simulink model "system_model"  (R2024a)
settings: Solver=VariableStepAuto  StartTime=0.0  StopTime=100000.0  MaxStep=1  RelTol=1e-9
values from neighbouring files (symbols this model uses):
  a_leader = 500*10^3 + earth_radi    (= 6871000)    [main.m]    (also in main_2.m)
  B_f_max = (C_d*A_f_max)/m_f    (= 0.78)    [main_2.m]
  B_f_min = (C_d*A_f_min)/m_f    (= 0.13)    [main_2.m]
  B_l_max = (C_d*A_l_max)/m_l    (= 0.78)    [main_2.m]
  B_l_min = (C_d*A_l_min)/m_l    (= 0.13)    [main_2.m]
  earth_radi = 6371*10^3    (= 6371000)    [main.m]    (also in main_2.m)
  J = eye(3)    [attitude.m]    (also in state_func.m = 43943563035.8; state_func_test.m = J_2 * R_E^2)
  J_2 = 1.08263 * 10^(-3)    (= 0.00108263)    [main.m]    (also in main_2.m; state_func.m)
  Kd = 5    [attitude.m]
  Kp = 5    [attitude.m]
  m_f = 1    [main.m]    (also in main_2.m = 2)
  m_l = 1    [main.m]    (also in main_2.m = 2)
  mu = 13/ 26.98    (= 0.481838398814)    [drag_coefficent_ruff_estimation.m]    (also in main.m = 6.67e-11; main_2.m = 398589196000000; state_func.m = 398589196000000; untitled5.m)
  q_0 = q_0 /norm(q_0)    [attitude.m]
  rho_leader = mean_rho_500km    (= 7.3e-13)    [main_2.m]
  w_0 = [1; 2; 1]    [attitude.m]
  x = theta_vec    [drag_coefficent_ruff_estimation.m]    (also in main.m = [d_a; d_lambda; d_e_x; d_e_y; d_i_x; d_i_y; d_Ballistic]; main_2.m = [d_a; d_lambda; d_e_x; d_e_y; d_i_x; d_i_y])
  x_f_prop = [a_follower; m_follower; e_follower; omega_follower; Omega_follower; i_follower]    [main_2.m]
  x_l_prop = [a_leader; m_leader; e_leader; omega_leader; Omega_leader; i_leader]    [main_2.m]
libraries: mpclib x1, slpidlib x1
(part 2 of 2)

== matlab function system_model/orbit_Propegation/MATLAB Function5 ==
  data: oeosc input; oemean output; j2 input; req input
function oemean = osc2mean (oeosc, j2, req)

% convert osculating classical orbital elements
% to mean classical orbital elements

% input

%  oeosc(1) = osculating semimajor axis (kilometers)
%  oeosc(2) = osculating orbital eccentricity (non-dimensional)
%             (0 <= eccentricity < 1)
%  oeosc(3) = osculating orbital inclination (radians)
%             (0 <= inclination <= pi)
%  oeosc(4) = osculating argument of perigee (radians)
%             (0 <= argument of perigee <= 2 pi)
%  oeosc(5) = osculating right ascension of ascending node (radians)
%             (0 <= raan <= 2 pi)
%  oeosc(6) = osculating true anomaly (radians)
%             (0 <= true anomaly <= 2 pi)

% output

%  oemean(1) = mean semimajor axis (kilometers)
%  oemean(2) = mean orbital eccentricity (non-dimensional)
%              (0 <= eccentricity < 1)
%  oemean(3) = mean orbital inclination (radians)
%              (0 <= inclination <= pi)
%  oemean(4) = mean argument of perigee (radians)
%              (0 <= argument of perigee <= 2 pi)
%  oemean(5) = mean right ascension of ascending node (radians)
%              (0 <= raan <= 2 pi)
%  oemean(6) = mean true anomaly (radians)
%              (0 <= true anomaly <= 2 pi)

% Orbital Mechanics with MATLAB

%%%%%%%%%%%%%%%%%%%%%%%%%%%%%%%

%global req j2

pi2 = 2.0 * pi;

oetmp = zeros(6, 1);

for i = 1:1:6
    
    oetmp(i) = oeosc(i);
    
end

a = sin(oetmp(6)) * sqrt(1.0 - oetmp(2) * oetmp(2));

b = oetmp(2) + cos(oetmp(6));

% eccentric anomaly

eanom = atan3(a, b);

% mean anomaly

oetmp(6) = mod(eanom - oetmp(2) * sin(eanom), pi2);

aos = oetmp(1);
eos = oetmp(2);
ios = oetmp(3);
apos = oetmp(4);
ranos = oetmp(5);
maos = oetmp(6);

aa = 1.0 / 3.0 - 0.5 * sin(ios)^2;

bb = 0.5 * sin(ios)^2;

if (eos < 0.01)
    
    lamos = mod(maos + apos, pi2);
    
    zos = eos * cos(apos);
    
    etaos = eos * sin(apos);
    
    sl = sin(lamos);
    cl = cos(lamos);
    
    s2l = sin(2 * lamos);
    c2l = cos(2 * lamos);
    
    s3l = sin(3 * lamos);
    c3l = cos(3 * lamos);
    
    s4l = sin(4 * lamos);
    c4l = cos(4 * lamos);
    
    s2i = sin(2 * ios);
    
    ci = cos(ios);
    
    am = aos;
    im = ios;
    ranm = ranos;
    mam = maos;
    lamm = lamos;
    zm = zos;
    etam = etaos;
    
    for n = 1:1:5
        
        asp = 3 * j2 * req * req / am * (bb * c2l + (1 - 3.5 * bb) ...
            * zm * cl + (1 - 2.5 * bb) * etam * sl + 3.5 * bb ...
            * (zm * c3l + etam * s3l));
        
        am = aos-asp;
        
        isp = 3 * j2 / 8 * req * req / am^2 * s2i * (c2l - zm * cl ...
            + etam * sl + 7/3 * (zm * c3l + etam * s3l));
        
        im = ios - isp;
        
        ci = cos(im);
        
        s2i = sin(2 * im);
        
        bb = 0.5 * sin(im)^2;
        
        ransp = 1.5 * j2 * req * req / am^2 * ci ...
            * (0.5 * s2l - 3.5 * zm * sl + 2.5 * etam * cl ...
            + 7/6 * (zm * s3l - etam * c3l));
        
        ranm = ranos - ransp;
        
        lamsp = 1.5 * j2 * req * req / (am * am) ...
            * (-0.5 * (1 - 5 * bb) * s2l + (7 - 77/4 * bb) ...
            * zm * sl - (6 - 55/4 * bb) * etam * cl - (7/6 - 77/12 * bb) ...
            * (zm * s3l - etam * c3l));
        
        lamm = lamos - lamsp;
        
        sl = sin(lamm);
        cl = cos(lamm);
        s2l = sin(2*lamm);
        c2l = cos(2*lamm);
        s3l = sin(3*lamm);
        c3l = cos(3*lamm);
        s4l = sin(4*lamm);
        c4l = cos(4*lamm);
        
        zsp = 1.5 * j2 * req * req / am^2 * ((1 - 2.5 * bb) * cl ...
            + 7/6 * bb * c3l + (1.5 - 5 * bb) * zm * c2l + (2 - 3 * bb) ...
            * etam * s2l + 17/4 * bb * (zm * c4l + etam * s4l));
        
        zm = zos - zsp;
        
        etasp = 1.5 * j2 * req * req / am^2 * ((1 - 3.5 * bb) * sl ...
            + 7/6 * bb * s3l + (1 - 6 * bb) * zm * s2l - (1.5 - 4 * bb) ...
            * etam * c2l + 17/4 * bb * (zm * s4l - etam * c4l));
        
        etam = etaos - etasp;
    end
    
    em = sqrt(etam^2 + zm^2);
    
    apm = 0;
    
    if (em > 1.0e-8)
        
        apm = atan2(etam, zm);
        
    end
    
    % "mean" mean anomaly
    
    mam = mod(lamm - apm, pi2);
    
else
    
    pm = aos*(1-eos^2);
    am = aos;
    em = eos;
    im = ios;
    apm = apos;
    ranm = ranos;
    mam = maos;
    
    [~, tam] = kepler1(mam, em);
    
    um = mod(apm+tam, pi2);
    
    hm = pm/(1+em*cos(tam));
    
    for n = 1:1:5
        
        asp = 3*j2*req*req/am*((am/hm)^3*(aa+bb*cos(2*um)) ...
            -aa*(1-em^2)^(-1.5));
        
        am = aos-asp;
        
        isp = 3/8*j2*req^2/pm^2*sin(2*im)*(cos(2*um) ...
            +em*cos(tam+2*apm)+1/3*em*cos(3*tam+2*apm));
        
        im = ios-isp;
        
        aa = 1/3-0.5*sin(im)^2;
        
        bb = 0.5*sin(im)^2;
        
        esp = 1.5*j2*req*req/am^2*((1-em^2)/em*((am/hm)^3 ...
            *(aa+bb*cos(2*um))-aa*(1-em^2)^(-1.5))-bb/(em*(1-em^2)) ...
            *(cos(2*um)+em*cos(tam+2*apm)+em*cos(3*tam+2.*apm)/3));
        
        em = eos-esp;
        
        pm = am * (1.0 - em^2);
        
        hm = pm / (1.0 + em * cos(tam));
        
        tam = mod(tam, 2.0 * pi);
        
        mam = mod(mam, 2.0 * pi);
        
        if ((abs(tam-pi) <= 1.0e-06) || (abs(mam-pi) <= 1.0e-06) || ...
                (abs(tam) <= 1.0e-06) || (abs(mam) <= 1.0e-06))
            
            eqoc = 0;
            
        else
            
            eqoc = tam-mam;
            
        end
        
        ransp = -1.5*j2*(req/pm)^2*cos(im)*(eqoc+em*sin(tam) ...
            -0.5*sin(2*um)-0.5*em*sin(tam+2*apm)-1/6*em*sin(3*tam+2*apm));
        
        ranm = ranos-ransp;
        
        apsp = 1.5*j2*(req/pm)^2*((2-5*bb)*(eqoc+em*sin(tam)) ...
            +(1-3*bb)*((1-0.25*em*em)*sin(tam)/em+0.5*sin(2*tam) ...
            +em*sin(3*tam)/12)-(0.5*bb+(0.5-15/8*bb)*em^2)/em*sin(tam+2*apm) ...
            +em/8*bb*sin(tam-2*apm)-0.5*(1-5*bb)*sin(2*um)+(7/6*bb ...
            -1/6*em^2*(1-19/4*bb))/em*sin(3*tam+2*apm) ...
            +0.75*bb*sin(4*tam+2*apm)+em/8*bb*sin(5*tam+2*apm));
        
        apm = apos-apsp;
        
        masp = 1.5*j2*(req/pm)^2*sqrt(1-em^2)/em*(-(1-3*bb)*((1-em^2/4) ...
            *sin(tam)+em/2*sin(2*tam)+em^2/12*sin(3*tam)) ...
            +bb*(0.5*(1+1.25*em^2)*sin(tam+2*apm)-em^2/8*sin(tam-2*apm) ...
            -7/6*(1-em^2/28)*sin(3*tam+2*apm)-0.75*em*sin(4*tam+2*apm) ...
            -em^2/8*sin(5*tam+2*apm)));
        
        mam = maos-masp;
        
        [~, tam] = kepler1(mam, em);
        
        um = mod(apm + tam, pi2);
    end
end
oemean = zeros(7,1);
oemean(1) = am;
oemean(2) = em;
oemean(3) = im;
oemean(4) = mod(apm, pi2);
oemean(5) = mod(ranm, pi2);
oemean(6) = mod(mam, pi2);

[~, ta] = kepler1(oemean(6), em);

oemean(7) = ta;


end

function y = atan3 (a, b)

% four quadrant inverse tangent

% input

%  a = sine of angle
%  b = cosine of angle

% output

%  y = angle (radians; 0 =< c <= 2 * pi)

% Orbital Mechanics with MATLAB

%%%%%%%%%%%%%%%%%%%%%%%%%%%%%%%

epsilon = 0.0000000001;

pidiv2 = 0.5 * pi;

if (abs(a) < epsilon)
    y = (1 - sign(b)) * pidiv2;
    return;
else
    c = (2 - sign(a)) * pidiv2;
end

if (abs(b) < epsilon)
    y = c;
    return;
else
    y = c + sign(a) * sign(b) * (abs(atan(a / b)) - pidiv2);
end

end

function [eanom, tanom] = kepler1 (manom, ecc)

% solve Kepler's equation for circular,
% elliptic and hyperbolic orbits

% Danby's method

% input

%  manom = mean anomaly (radians)
%  ecc   = orbital eccentricity (non-dimensional)

% output

%  eanom = eccentric anomaly (radians)
%  tanom = true anomaly (radians)

% Orbital Mechanics with MATLAB

%%%%%%%%%%%%%%%%%%%%%%%%%%%%%%%

%global  niter

% define convergence criterion

ktol = 1.0e-10;

pi2 = 2.0 * pi;

xma = manom - pi2 * fix(manom/pi2);

% initial guess

if (ecc == 0.0)
    
    % circular orbit

    tanom = xma;
    eanom = xma;
    return;
    
elseif (ecc < 1.0)
    % elliptic orbit

    eanom = xma + 0.85 * sign(sin(xma)) * ecc;

else
    % hyperbolic orbit

    eanom = log(2.0 * xma / ecc + 1.8);
end

% perform iterations

niter = 0;

while(1)
    
    if (ecc < 1)

        % elliptic orbit

        s = ecc * sin(eanom);
        c = ecc * cos(eanom);

        f = eanom - s - xma;
        fp = 1 - c;
        fpp = s;
        fppp = c;
        
    else

        % hyperbolic orbit

        s = ecc * sinh(eanom);
        c = ecc * cosh(eanom);

        f = s - eanom - xma;
        fp = c - 1;
        fpp = s;
        fppp = c;
        
    end

    niter = niter + 1;

    % check for convergence

    if (abs(f) <= ktol || niter > 20)
        
        break;
        
    end

    % update eccentric anomaly

    delta = -f / fp;

    deltastar = -f / (fp + 0.5 * delta * fpp);

    deltak = -f / (fp + 0.5 * deltastar * fpp ...
        + deltastar * deltastar * fppp / 6);

    eanom = eanom + deltak;
end

if (niter > 20)
    
    %clc; home;
    
    fprintf('\n\n   more than 20 iterations in kepler1 \n\n');
    
    %pause;
    
    %return;
end

% compute true anomaly

if (ecc < 1)
    % elliptic orbit

    sta = sqrt(1 - ecc * ecc) * sin(eanom);
    cta = cos(eanom) - ecc;
else
    % hyperbolic orbit

    sta = sqrt(ecc * ecc - 1) * sinh(eanom);
    cta = ecc - cosh(eanom);
end

tanom = atan3(sta, cta);


end

== matlab function system_model/g(x) ==
  data: u input; x input; g_x output; x_f input; rho input
function g_x = g(u, x, x_f, rho)
%Note that these equations have elliminated the need for leader spacecraft
%orbit properties

B   = u(1);
B_f = u(2);

rho_c = rho;


a_c = x_f(1);
%u_c = x_f(2);
e_c = x_f(2);
% e_c = x_f(3); - not corrrect here
%i_c = x_f(4);  - not correct here
i_c = x_f(3);
omega_c = x_f(4);
Omega_c = x_f(5);
Nu_c    = x_f(6);
%  oemean(1) = mean semimajor axis (kilometers)
%  oemean(2) = mean orbital eccentricity (non-dimensional)
%              (0 <= eccentricity < 1)
%  oemean(3) = mean orbital inclination (radians)
%              (0 <= inclination <= pi)
%  oemean(4) = mean argument of perigee (radians)
%              (0 <= argument of perigee <= 2 pi)
%  oemean(5) = mean right ascension of ascending node (radians)
%              (0 <= raan <= 2 pi)
%  oemean(6) = mean true anomaly (radians)
%              (0 <= true anomaly <= 2 pi)
%x_f = [a_dot; M_dot; e_dot; omega_dot; Omega_dot; i_dot];

betta   = B*f(e_c)*rho;
betta_c = B_f *f(e_c) * rho_c;
E       = sqrt(e_c^2 + x(3)^2 + x(4)^2 - 2*e_c*(x(3)*cos(omega_c) + x(4)*sin(omega_c)));



g_x = zeros(6,1);

g_x(1) = (1 + x(1))*(betta_c/(1-e_c) + betta/(E-1) );
g_x(2) = 0;
g_x(3) = betta_c * cos(omega_c) + E^-1 * betta*( x(3) - e_c*cos(omega_c));
g_x(4) = betta_c * sin(omega_c) + E^-1 * betta*( x(4) - e_c*sin(omega_c));
g_x(5) = 0;
g_x(6) = 0;

end
     
function f = f(e)
    f = 1.61*10^4*e^0.02701 -1.61*10^4;
end

== matlab function system_model/orbit_Propegation/MATLAB Function6 ==
  data: xn output; x input
function xn = kozsak(x)

iflag = 2;

% convert between osculating and mean classical orbital elements

% method due to Chauncey Uphoff (JPL IOM 312/85.2-927)

% input

%  iflag = 1 => mean to osculating
%          2 => osculating to mean

%  x = osculating or mean orbital elements

% output

%  xn = osculating or mean orbital elements

% Orbital Mechanics with MATLAB

%%%%%%%%%%%%%%%%%%%%%%%%%%%%%%%

pi2 = 2.0 * pi;

xi = zeros(6, 1);

xn = zeros(6, 1);

% set max iterations based on input orbital eccentricity x(2)

if (x(2) < 0.1)
    
    imax = 10;
    
elseif (x(2) < 0.01)
    
    imax = 20;
    
elseif (x(2) < 0.001)
    
    imax = 30;
    
else
    
    imax = 5;
    
end

for i = 1:1:6
    
    xi(i) = x(i);
    
end

icount = 0;

while (1)
    
    % compute periodics
    
    dx = delm(x);
    
    if (iflag == 2)
        
        % osculating to mean
        
        icount = icount + 1;
        
        for i = 1:1:6
            
            xn(i) = xi(i) - dx(i);
            
        end
        
        % check for negative eccentricity
        
        if (xn(2) < 0.0)
            
            xn(2) = 0.0;
            
        end
        
        for i = 3:1:6
            
            xn(i) = mod(xn(i) + pi2, pi2);
            
        end
        
        % check for maximum iterations
        
        if (icount == imax)
            
            break;
            
        end
        
        % load mean orbital elements
        
        for i = 1:1:6
            
            x(i) = xn(i);
            
        end
        
    else
        
        % mean to osculating
        
        for i = 1:1:6
            
            xn(i) = xi(i) + dx(i);
            
        end
        
        for i = 3:1:6
            
            xn(i) = mod(xn(i) + pi2, pi2);
            
        end
        
        break;
        
    end
    
end

end

function dx = delm (x)

% compute [osculating - mean] classical orbital elements

% input

%  x = mean classical orbital elements

% output

%  dx = [osculating - mean] classical orbital elements

% Orbital Mechanics with MATLAB

%%%%%%%%%%%%%%%%%%%%%%%%%%%%%%%

mu  = 98600.4415;
req = 6378.14;
xj2 = 0.001082634;

pi2 = 2.0 * pi;

dx = zeros(6, 1);

% semimajor axis (kilometers)

a = x(1);

% orbital eccentricity (non-dimensional)

e = x(2);

% orbital inclination (radians)

ai = x(3);

% right ascension of the ascending node (radians)

an = x(4);

% argument of perigee (radians)

w = x(5);

% mean anomaly (radians)

am = x(6);

% compute true anomaly from mean anomaly

f = anomly(2, am, e);

f = mod(f + pi2, pi2);

am = mod(am + pi2, pi2);

si = sin(ai);
ci = cos(ai);
ti = si / ci;

si2 = si * si;
ci2 = ci * ci;

sf = sin(f);
cf = cos(f);
s2f = sin(2.0 * f);

u = f + w;
e2 = e * e;
esf = e * sf;

d1 = 1.0 - e2;
d2 = sqrt(d1);
d3 = e * cf;
d4 = 1.0 + d3;
d42 = d4 * d4;
d5 = 1.0 + d2;
d6 = (3.0 * ci2 - 1.0) / d5;

p = a * d1;

d7 = sqrt(mu / p);

r = p / d4;

rdot = d7 * esf;

twou = 2.0 * u;

twow = 2.0 * w;

s2u = sin(twou);
c2u = cos(twou);

sf2w = sin(f + twow);

d8 = 3.0 * f + twow;

s3f2w = sin(d8);
cf2w = cos(f + twow);
c3f2w = cos(d8);

q1 = xj2 * (req / p) ^ 2;

di = 0.75 * q1 * si * ci * (c2u + e * cf2w + e / 3.0 * c3f2w);

dp = 2.0 * p * ti * di;

dummy1 = f - am + esf - 0.5 * s2u - 0.5 * e * sf2w - e * s3f2w / 6.0;

dn = -1.5 * q1 * ci * dummy1;

dr = -0.25 * p * q1 * ((3.0 * ci2 - 1.0) * (2.0 * d2 / d4 + d3 / d5 + 1.0) - si2 * c2u);

drdot = 0.25 * d7 * q1 * (d6 * esf * (d2 * d5 + d42) - 2.0 * si2 * d42 * s2u);

du = -0.125 * q1 * (6.0 * (1.0 - 5.0 * ci2) * (f - am) + 4.0 * esf * ((1.0 - 6.0 * ci2) ...
    - d6) - d6 * e2 * s2f + 2.0 * (5.0 * ci2 - 2.0) * e * sf2w + (7.0 * ci2 - 1.0) ...
    * s2u + 2.0 * ci2 * e * s3f2w);

pnw = p + dp;

ainw = ai + di;

annw = an + dn;

rnw = r + dr;

rdotnw = rdot + drdot;

unw = u + du;

aa = pnw / rnw - 1.0;

bb = sqrt(pnw / mu) * rdotnw;

enw2 = aa * aa + bb * bb;

enw = sqrt(enw2);

fnw = atan2(bb, aa);

anw = pnw / (1.0 - enw2);

wnw = unw - fnw;

amnw = anomly(5, fnw, enw);

%  compute [osculating - mean] classical orbital elements

dx(1) = anw - a;

dx(2) = enw - e;

dx(3) = ainw - ai;

dx(4) = annw - an;

dx(5) = wnw - w;

dx(6) = amnw - am;

end

function aout = anomly(nflag, ain, ecc)

% orbital anomaly function

% input

%  nflag = 1 => mean to eccentric
%          2 => mean to true
%          3 => eccentric to mean
%          4 => eccentric to true
%          5 => true to mean
%          6 => true to eccentric

%  ain = input anomaly (radians)
%  ecc = orbital eccentricity

% output

%  aout = output anomaly (radians)

% Orbital Mechanics with MATLAB

%%%%%%%%%%%%%%%%%%%%%%%%%%%%%%%

switch nflag
    
    case {1, 2}
        
        % mean anomaly
        
        am = ain;
        
    case {3, 4}
        
        % eccentric anomaly
        
        ea = ain;
        
    case {5, 6}
        
        % true anomaly
        
        f = ain;
        
end

if (nflag == 1 || nflag == 2)
    
    % eccentric anomaly (radians)
    
    ea = kepler(am, ecc);
    
end

if (nflag == 2 || nflag == 4)
    
    % true anomaly (radians)
    
    f = 2.0 * atan(sqrt((1.0 + ecc) / (1.0 - ecc)) * tan(ea / 2.0));
    
end

if (nflag == 5 || nflag == 6)
    
    % eccentric anomaly (radians)
    
    ea = 2.0 * atan(sqrt((1.0 - ecc) / (1.0 + ecc)) * tan(f / 2.0));
    
end

if (nflag == 5 || nflag == 3)
    
    % mean anomaly (radians)
    
    am = ea - ecc * sin(ea);
    
end

switch nflag
    
    case {1, 6}
        
        % eccentric anomaly
        
        aout = ea;
        
    case {2, 4}
        
        % true anomaly
        
        aout = f;
        
    case {3, 5}
        
        % mean anomaly
        
        aout = am;
end
end


function eanom = kepler(manom, ecc)

% solve Kepler's equation for circular,
% elliptic and hyperbolic orbits

% Danby's method

% input

%  manom = mean anomaly (radians)
%  ecc   = orbital eccentricity (non-dimensional)

% output

%  eanom = eccentric anomaly (radians)

% Orbital Mechanics with MATLAB

%%%%%%%%%%%%%%%%%%%%%%%%%%%%%%%

% define convergence criterion

ktol = 1.0e-10;

pi2 = 2.0 * pi;

xma = manom - pi2 * fix(manom/pi2);

% initial guess

if (ecc == 0.0)
    
    % circular orbit
    
    eanom = xma;
    
    return;
    
elseif (ecc < 1.0)
    
    % elliptic orbit

    eanom = xma + 0.85 * sign(sin(xma)) * ecc;

else
    
    % hyperbolic orbit

    eanom = log(2.0 * xma / ecc + 1.8);
    
end

% perform iterations

niter = 0;

while(1)
    
    if (ecc < 1.0)

        % elliptic orbit

        s = ecc * sin(eanom);
        c = ecc * cos(eanom);

        f = eanom - s - xma;
        fp = 1.0 - c;
        fpp = s;
        fppp = c;
        
    else

        % hyperbolic orbit

        s = ecc * sinh(eanom);
        c = ecc * cosh(eanom);

        f = s - eanom - xma;
        fp = c - 1.0;
        fpp = s;
        fppp = c;
        
    end

    niter = niter + 1;

    % check for convergence

    if (abs(f) <= ktol || niter > 20)
        
        break;
        
    end

    % update eccentric anomaly

    delta = -f / fp;

    deltastar = -f / (fp + 0.5 * delta * fpp);

    deltak = -f / (fp + 0.5 * deltastar * fpp ...
        + deltastar * deltastar * fppp / 6.0);

    eanom = eanom + deltak;
    
end

if (niter > 20)
    
    fprintf('\n\n   more than 20 iterations in kepler \n\n');

end






end

== matlab function system_model/orbit_Propegation/MATLAB Function7 ==
  data: x_f input; x_l input; d_a output; d_lambda output; d_e_x output; d_e_y output; d_i_x output; d_i_y output
function [d_a, d_lambda, d_e_x, d_e_y, d_i_x, d_i_y] = toRelOribtialElements(x_f, x_l)


a_f     = x_f(1);
e_f     = x_f(2);
i_f     = x_f(3);
omega_f = x_f(4);
Omega_f = x_f(5);
M_f     = x_f(6);

a_l     = x_l(1);
e_l     = x_l(2);
i_l     = x_l(3);
omega_l = x_l(4);
Omega_l = x_l(5);
M_l     = x_l(6);



u_l    = omega_l + M_l;
u_f    = omega_f + M_f;
u_diff =  ssa(M_f -M_l) + ssa(omega_f - omega_l); 

d_a          = (a_f - a_l) / a_l;
%d_lambda     = (u_f - u_l) + (Omega_f - Omega_l)*cos(i_l);
d_lambda     = u_diff + (Omega_f - Omega_l)*cos(i_l);
d_e_x        = e_f*cos(omega_f) - e_l*cos(omega_l);
d_e_y        = e_f*sin(omega_f) - e_l*sin(omega_l);
d_i_x        = i_f - i_l;
d_i_y        = (Omega_f -Omega_l)*sin(i_l);


end

function angle = ssa(angle)
    angle = mod( angle + pi, 2 * pi ) - pi; 
end

== matlab function system_model/orbit_Propegation/MATLAB Function8 ==
  data: oeosc input; oemean output; j2 input; req input
function oemean = osc2mean (oeosc, j2, req)

% convert osculating classical orbital elements
% to mean classical orbital elements

% input

%  oeosc(1) = osculating semimajor axis (kilometers)
%  oeosc(2) = osculating orbital eccentricity (non-dimensional)
%             (0 <= eccentricity < 1)
%  oeosc(3) = osculating orbital inclination (radians)
%             (0 <= inclination <= pi)
%  oeosc(4) = osculating argument of perigee (radians)
%             (0 <= argument of perigee <= 2 pi)
%  oeosc(5) = osculating right ascension of ascending node (radians)
%             (0 <= raan <= 2 pi)
%  oeosc(6) = osculating true anomaly (radians)
%             (0 <= true anomaly <= 2 pi)

% output

%  oemean(1) = mean semimajor axis (kilometers)
%  oemean(2) = mean orbital eccentricity (non-dimensional)
%              (0 <= eccentricity < 1)
%  oemean(3) = mean orbital inclination (radians)
%              (0 <= inclination <= pi)
%  oemean(4) = mean argument of perigee (radians)
%              (0 <= argument of perigee <= 2 pi)
%  oemean(5) = mean right ascension of ascending node (radians)
%              (0 <= raan <= 2 pi)
%  oemean(6) = mean true anomaly (radians)
%              (0 <= true anomaly <= 2 pi)

% Orbital Mechanics with MATLAB

%%%%%%%%%%%%%%%%%%%%%%%%%%%%%%%

%global req j2

pi2 = 2.0 * pi;

oetmp = zeros(6, 1);

for i = 1:1:6
    
    oetmp(i) = oeosc(i);
    
end

a = sin(oetmp(6)) * sqrt(1.0 - oetmp(2) * oetmp(2));

b = oetmp(2) + cos(oetmp(6));

% eccentric anomaly

eanom = atan3(a, b);

% mean anomaly

oetmp(6) = mod(eanom - oetmp(2) * sin(eanom), pi2);

aos = oetmp(1);
eos = oetmp(2);
ios = oetmp(3);
apos = oetmp(4);
ranos = oetmp(5);
maos = oetmp(6);

aa = 1.0 / 3.0 - 0.5 * sin(ios)^2;

bb = 0.5 * sin(ios)^2;

if (eos < 0.01)
    
    lamos = mod(maos + apos, pi2);
    
    zos = eos * cos(apos);
    
    etaos = eos * sin(apos);
    
    sl = sin(lamos);
    cl = cos(lamos);
    
    s2l = sin(2 * lamos);
    c2l = cos(2 * lamos);
    
    s3l = sin(3 * lamos);
    c3l = cos(3 * lamos);
    
    s4l = sin(4 * lamos);
    c4l = cos(4 * lamos);
    
    s2i = sin(2 * ios);
    
    ci = cos(ios);
    
    am = aos;
    im = ios;
    ranm = ranos;
    mam = maos;
    lamm = lamos;
    zm = zos;
    etam = etaos;
    
    for n = 1:1:5
        
        asp = 3 * j2 * req * req / am * (bb * c2l + (1 - 3.5 * bb) ...
            * zm * cl + (1 - 2.5 * bb) * etam * sl + 3.5 * bb ...
            * (zm * c3l + etam * s3l));
        
        am = aos-asp;
        
        isp = 3 * j2 / 8 * req * req / am^2 * s2i * (c2l - zm * cl ...
            + etam * sl + 7/3 * (zm * c3l + etam * s3l));
        
        im = ios - isp;
        
        ci = cos(im);
        
        s2i = sin(2 * im);
        
        bb = 0.5 * sin(im)^2;
        
        ransp = 1.5 * j2 * req * req / am^2 * ci ...
            * (0.5 * s2l - 3.5 * zm * sl + 2.5 * etam * cl ...
            + 7/6 * (zm * s3l - etam * c3l));
        
        ranm = ranos - ransp;
        
        lamsp = 1.5 * j2 * req * req / (am * am) ...
            * (-0.5 * (1 - 5 * bb) * s2l + (7 - 77/4 * bb) ...
            * zm * sl - (6 - 55/4 * bb) * etam * cl - (7/6 - 77/12 * bb) ...
            * (zm * s3l - etam * c3l));
        
        lamm = lamos - lamsp;
        
        sl = sin(lamm);
        cl = cos(lamm);
        s2l = sin(2*lamm);
        c2l = cos(2*lamm);
        s3l = sin(3*lamm);
        c3l = cos(3*lamm);
        s4l = sin(4*lamm);
        c4l = cos(4*lamm);
        
        zsp = 1.5 * j2 * req * req / am^2 * ((1 - 2.5 * bb) * cl ...
            + 7/6 * bb * c3l + (1.5 - 5 * bb) * zm * c2l + (2 - 3 * bb) ...
            * etam * s2l + 17/4 * bb * (zm * c4l + etam * s4l));
        
        zm = zos - zsp;
        
        etasp = 1.5 * j2 * req * req / am^2 * ((1 - 3.5 * bb) * sl ...
            + 7/6 * bb * s3l + (1 - 6 * bb) * zm * s2l - (1.5 - 4 * bb) ...
            * etam * c2l + 17/4 * bb * (zm * s4l - etam * c4l));
        
        etam = etaos - etasp;
    end
    
    em = sqrt(etam^2 + zm^2);
    
    apm = 0;
    
    if (em > 1.0e-8)
        
        apm = atan2(etam, zm);
        
    end
    
    % "mean" mean anomaly
    
    mam = mod(lamm - apm, pi2);
    
else
    
    pm = aos*(1-eos^2);
    am = aos;
    em = eos;
    im = ios;
    apm = apos;
    ranm = ranos;
    mam = maos;
    
    [~, tam] = kepler1(mam, em);
    
    um = mod(apm+tam, pi2);
    
    hm = pm/(1+em*cos(tam));
    
    for n = 1:1:5
        
        asp = 3*j2*req*req/am*((am/hm)^3*(aa+bb*cos(2*um)) ...
            -aa*(1-em^2)^(-1.5));
        
        am = aos-asp;
        
        isp = 3/8*j2*req^2/pm^2*sin(2*im)*(cos(2*um) ...
            +em*cos(tam+2*apm)+1/3*em*cos(3*tam+2*apm));
        
        im = ios-isp;
        
        aa = 1/3-0.5*sin(im)^2;
        
        bb = 0.5*sin(im)^2;
        
        esp = 1.5*j2*req*req/am^2*((1-em^2)/em*((am/hm)^3 ...
            *(aa+bb*cos(2*um))-aa*(1-em^2)^(-1.5))-bb/(em*(1-em^2)) ...
            *(cos(2*um)+em*cos(tam+2*apm)+em*cos(3*tam+2.*apm)/3));
        
        em = eos-esp;
        
        pm = am * (1.0 - em^2);
        
        hm = pm / (1.0 + em * cos(tam));
        
        tam = mod(tam, 2.0 * pi);
        
        mam = mod(mam, 2.0 * pi);
        
        if ((abs(tam-pi) <= 1.0e-06) || (abs(mam-pi) <= 1.0e-06) || ...
                (abs(tam) <= 1.0e-06) || (abs(mam) <= 1.0e-06))
            
            eqoc = 0;
            
        else
            
            eqoc = tam-mam;
            
        end
        
        ransp = -1.5*j2*(req/pm)^2*cos(im)*(eqoc+em*sin(tam) ...
            -0.5*sin(2*um)-0.5*em*sin(tam+2*apm)-1/6*em*sin(3*tam+2*apm));
        
        ranm = ranos-ransp;
        
        apsp = 1.5*j2*(req/pm)^2*((2-5*bb)*(eqoc+em*sin(tam)) ...
            +(1-3*bb)*((1-0.25*em*em)*sin(tam)/em+0.5*sin(2*tam) ...
            +em*sin(3*tam)/12)-(0.5*bb+(0.5-15/8*bb)*em^2)/em*sin(tam+2*apm) ...
            +em/8*bb*sin(tam-2*apm)-0.5*(1-5*bb)*sin(2*um)+(7/6*bb ...
            -1/6*em^2*(1-19/4*bb))/em*sin(3*tam+2*apm) ...
            +0.75*bb*sin(4*tam+2*apm)+em/8*bb*sin(5*tam+2*apm));
        
        apm = apos-apsp;
        
        masp = 1.5*j2*(req/pm)^2*sqrt(1-em^2)/em*(-(1-3*bb)*((1-em^2/4) ...
            *sin(tam)+em/2*sin(2*tam)+em^2/12*sin(3*tam)) ...
            +bb*(0.5*(1+1.25*em^2)*sin(tam+2*apm)-em^2/8*sin(tam-2*apm) ...
            -7/6*(1-em^2/28)*sin(3*tam+2*apm)-0.75*em*sin(4*tam+2*apm) ...
            -em^2/8*sin(5*tam+2*apm)));
        
        mam = maos-masp;
        
        [~, tam] = kepler1(mam, em);
        
        um = mod(apm + tam, pi2);
    end
end
oemean = zeros(7,1);
oemean(1) = am;
oemean(2) = em;
oemean(3) = im;
oemean(4) = mod(apm, pi2);
oemean(5) = mod(ranm, pi2);
oemean(6) = mod(mam, pi2);

[~, ta] = kepler1(oemean(6), em);

oemean(7) = ta;


end

function y = atan3 (a, b)

% four quadrant inverse tangent

% input

%  a = sine of angle
%  b = cosine of angle

% output

%  y = angle (radians; 0 =< c <= 2 * pi)

% Orbital Mechanics with MATLAB

%%%%%%%%%%%%%%%%%%%%%%%%%%%%%%%

epsilon = 0.0000000001;

pidiv2 = 0.5 * pi;

if (abs(a) < epsilon)
    y = (1 - sign(b)) * pidiv2;
    return;
else
    c = (2 - sign(a)) * pidiv2;
end

if (abs(b) < epsilon)
    y = c;
    return;
else
    y = c + sign(a) * sign(b) * (abs(atan(a / b)) - pidiv2);
end

end

function [eanom, tanom] = kepler1 (manom, ecc)

% solve Kepler's equation for circular,
% elliptic and hyperbolic orbits

% Danby's method

% input

%  manom = mean anomaly (radians)
%  ecc   = orbital eccentricity (non-dimensional)

% output

%  eanom = eccentric anomaly (radians)
%  tanom = true anomaly (radians)

% Orbital Mechanics with MATLAB

%%%%%%%%%%%%%%%%%%%%%%%%%%%%%%%

%global  niter

% define convergence criterion

ktol = 1.0e-10;

pi2 = 2.0 * pi;

xma = manom - pi2 * fix(manom/pi2);

% initial guess

if (ecc == 0.0)
    
    % circular orbit

    tanom = xma;
    eanom = xma;
    return;
    
elseif (ecc < 1.0)
    % elliptic orbit

    eanom = xma + 0.85 * sign(sin(xma)) * ecc;

else
    % hyperbolic orbit

    eanom = log(2.0 * xma / ecc + 1.8);
end

% perform iterations

niter = 0;

while(1)
    
    if (ecc < 1)

        % elliptic orbit

        s = ecc * sin(eanom);
        c = ecc * cos(eanom);

        f = eanom - s - xma;
        fp = 1 - c;
        fpp = s;
        fppp = c;
        
    else

        % hyperbolic orbit

        s = ecc * sinh(eanom);
        c = ecc * cosh(eanom);

        f = s - eanom - xma;
        fp = c - 1;
        fpp = s;
        fppp = c;
        
    end

    niter = niter + 1;

    % check for convergence

    if (abs(f) <= ktol || niter > 20)
        
        break;
        
    end

    % update eccentric anomaly

    delta = -f / fp;

    deltastar = -f / (fp + 0.5 * delta * fpp);

    deltak = -f / (fp + 0.5 * deltastar * fpp ...
        + deltastar * deltastar * fppp / 6);

    eanom = eanom + deltak;
end

if (niter > 20)
    
    %clc; home;
    
    fprintf('\n\n   more than 20 iterations in kepler1 \n\n');
    
    %pause;
    
    %return;
end

% compute true anomaly

if (ecc < 1)
    % elliptic orbit

    sta = sqrt(1 - ecc * ecc) * sin(eanom);
    cta = cos(eanom) - ecc;
else
    % hyperbolic orbit

    sta = sqrt(ecc * ecc - 1) * sinh(eanom);
    cta = ecc - cosh(eanom);
end

tanom = atan3(sta, cta);


end

== matlab function system_model/orbit_Propegation/MATLAB Function9 ==
  data: m input; B input; Cd output; theta input; A output
function [Cd, A] = fcn(m, B, theta)

    % B - Ballistic coefficent
    % theta - pitch angle of craft


    alpha = (7.5*10^(-17)*5.14*10^7*10^6*1011)/ (1.0 + (7.5*10^(-17)*5.14*10^7*10^6*1011)); % for NRLSMIE-00 model
    r = sqrt(1-alpha);

    %flat plate at incidence theta
    C_d_flat_theta = 2*(1+(2/3)*r*sin(theta));
    C_d_flat_theta_inv = 2*(1+(2/3)*r*sin(pi/2-theta));
    
    % portion of total area as A_ref, must be modified for spesific
    % spacecraft
    
    %Areas
    %2 solar panels
    A_tot_solar = 2*15*15;
    A_ref_solar = A_tot_solar*sin(theta);
    
    %box (front and upper side)
    A_tot_box_front = 10*10;
    A_tot_box_top   = 15*10;
    
    A_ref_box_front = A_tot_box_front*cos(theta);
    A_ref_box_top   = A_tot_box_top*sin(theta);
    
    A_ref_tot = A_ref_solar + A_ref_box_top + A_ref_box_front;
    
    %Total drag coefficent
    Cd = (A_ref_box_front/A_ref_tot)* C_d_flat_theta_inv + ((A_ref_tot-A_ref_box_front)/A_ref_tot)* C_d_flat_theta;
    A = (B*m)/ Cd;
    
end

== matlab function system_model/orbit_Propegation/MATLAB Function10 ==
  data: m input; B input; Cd output; theta input; A output
function [Cd, A] = fcn(m, B, theta)

    % B - Ballistic coefficent
    % theta - pitch angle of craft


    alpha = (7.5*10^(-17)*5.14*10^7*10^6*1011)/ (1.0 + (7.5*10^(-17)*5.14*10^7*10^6*1011)); % for NRLSMIE-00 model
    r = sqrt(1-alpha);

    %flat plate at incidence theta
    C_d_flat_theta = 2*(1+(2/3)*r*sin(theta));
    C_d_flat_theta_inv = 2*(1+(2/3)*r*sin(pi/2-theta));
    
    % portion of total area as A_ref, must be modified for spesific
    % spacecraft
    
    %Areas
    %2 solar panels
    A_tot_solar = 2*15*15;
    A_ref_solar = A_tot_solar*sin(theta);
    
    %box (front and upper side)
    A_tot_box_front = 10*10;
    A_tot_box_top   = 15*10;
    
    A_ref_box_front = A_tot_box_front*cos(theta);
    A_ref_box_top   = A_tot_box_top*sin(theta);
    
    A_ref_tot = A_ref_solar + A_ref_box_top + A_ref_box_front;
    
    %Total drag coefficent
    Cd = (A_ref_box_front/A_ref_tot)* C_d_flat_theta_inv + ((A_ref_tot-A_ref_box_front)/A_ref_tot)* C_d_flat_theta;
    A = (B*m)/ Cd;
    

end

== matlab function system_model/m ==
  data: x_f input; a_f_nmp output; e_f_nmp output; i_f_nmpc output; omega_f_nmpc output
function [a_f_nmp, e_f_nmp, i_f_nmpc, omega_f_nmpc] = fcn(x_f)

    a_f_nmp     = x_f(1);
    e_f_nmp     = x_f(2);
    i_f_nmpc     = x_f(3);
    omega_f_nmpc = x_f(4);

== matlab function system_model/m1 ==
  data: x_f input; a_f_nmp output
function a_f_nmp = fcn(x_f)

    a_f_nmp     = x_f(1);

== matlab function system_model/m2 ==
  data: x_f input; e_f_nmp output
function e_f_nmp = fcn(x_f)

    e_f_nmp     = x_f(2);

== matlab function system_model/m3 ==
  data: x_f input; i_f_nmpc output
function i_f_nmpc = fcn(x_f)

    i_f_nmpc     = x_f(3);

== matlab function system_model/m4 ==
  data: x_f input; omega_f_nmpc output
function omega_f_nmpc = fcn(x_f)

    omega_f_nmpc = x_f(4);

== matlab function system_model/orbit_Propegation/MATLAB Function11 ==
  data: ob_km input; ob_m output
function ob_m = km2m (ob_km)

% km to m in the orbital parameteres

ob_m = ob_km;
ob_m(1) = 10^3 * ob_km(1);

== matlab function system_model/orbit_Propegation/MATLAB Function12 ==
  data: ob_km input; ob_m output
function ob_m = km2m (ob_km)

% km to m in the orbital parameteres

ob_m = ob_km;
ob_m(1) = 10^3 * ob_km(1);

== matlab function system_model/f(x) ==
  data: x input; x_f input; f_x output; mu input; J_2 input; R_E input
function f_x = f(x, x_f, mu, J_2, R_E)
    
    a_c = x_f(1);
    %u_c = x_f(2);
    e_c = x_f(2);
    i_c = x_f(3);
    %  oemean(1) = mean semimajor axis (kilometers)
    %  oemean(2) = mean orbital eccentricity (non-dimensional)
    %              (0 <= eccentricity < 1)
    %  oemean(3) = mean orbital inclination (radians)
    %              (0 <= inclination <= pi)
    %  oemean(4) = mean argument of perigee (radians)
    %              (0 <= argument of perigee <= 2 pi)
    %  oemean(5) = mean right ascension of ascending node (radians)
    %              (0 <= raan <= 2 pi)
    %  oemean(6) = mean true anomaly (radians)
    %              (0 <= true anomaly <= 2 pi)


     A = (3/2) * sqrt( ( (1 + x(1))^7 *mu)/(a_c^7) );
     I = 3 + 5 *cos(2*(i_c - x(5)) );
     J       = J_2 * R_E^2;
    

     f_x = zeros(6,1);
     f_x(1) = 0;
     f_x(2) = -0.5 * A *( (2*(a_c^2)*x(1)) /(1 + x(1))^2 + 7 * J * sin( 2*( i_c - x(5) ) )*x(5) );
     f_x(3) = -0.25 * J * A *I * x(4);
     f_x(4) =  0.25 * J * A *I * x(3);
     f_x(5) = 0;
     f_x(6) = J * A * sin( i_c - x(5) )^2 * x(5); % possible bug here, should check equations

== matlab function system_model/orbit_Propegation/MATLAB Function13 ==
  data: ob_km input; ob_m output
function ob_m = km2m (ob_km)

% km to m in the orbital parameteres

ob_m = ob_km;
ob_m(1) = 10^3 * ob_km(1);

== matlab function system_model/orbit_Propegation/MATLAB Function ==
  data: r input; a output; v input; mu input; e output; i output; Omega output; omega output; nu output; M output
function [a, e, i, Omega, omega, nu, M] = cart2kep(r, v, mu)
% CART2KEP converts Cartesian coordinates to Keplerian orbital elements
% Input arguments:
% r   - position vector (km)
% v   - velocity vector (km/s)
% mu  - gravitational parameter (km^3/s^2)
% Output arguments:
% a     - semi-major axis (km)
% e     - eccentricity
% i     - inclination (rad)
% Omega - right ascension of the ascending node (rad)
% omega - argument of perigee (rad)
% E     - eccentric anomaly (rad)

% Compute specific angular momentum and its magnitude
h = cross(r, v);
hmag = norm(h);

% Compute semi-latus rectum and eccentricity
rp = hmag^2/mu;
evec = cross(v, h)/mu - r/norm(r);
e = norm(evec);

% Compute semi-major axis and true anomaly
%a = rp/(1-e^2);
a = 1/( (2/norm(r)-(norm(v)^2/mu)) );
cos_nu = dot(evec, r)/(e*norm(r));
sin_nu = dot(cross(r, v), h)/(e*norm(r)*hmag);
%nu = atan2(sin_nu, cos_nu);
nu = acos(dot(evec,r)/(e*norm(r)));

if dot(r,v)<0
   nu = 2*pi - nu;
end



%TEst
%nu_dot = hmag/norm(r)^2;



% Test that did not work well
%if dot(r,v)>0
%    nu = acos(cos_nu);
%else
%    nu = 0;%2*pi - acos(cos_nu);
%end

% Compute inclination and right ascension of the ascending node
i = acos(h(3)/hmag);
Omega = atan2(h(1), -h(2));

% Compute argument of perigee and eccentric anomaly
cos_omega = evec(1)/e;
sin_omega = evec(2)/e;
omega = atan2(sin_omega, cos_omega) - Omega;
%omega = atan2(sin_omega, cos_omega);

cos_E = (1 - norm(r)/a)/e;
sin_E = dot(r, v)/(e*norm(r));
E = atan2(sin_E, cos_E);

%mean anomally
%atan_y = (e+cos(nu));
%atan_x = (sqrt(1-e^2)*sin(nu));
%E = atan2(atan_x, atan_y);
%M = E - e*sin(E);

%Mean in python
 E = atan2(sqrt(1 - e^2) * sin(nu), e + cos(nu));
 E = mod(E, 2 * pi);
 M = E - e * sin(E);

%es = ((sqrt(1-e*e))*sin(E))./(1-e*cos(E));
%ec = (cos(E)-e)./(1-e*cos(E));
%nu = atan2(es,ec);
 % For elliptical orbits, iterative methods like universal variable method 
  % are needed for accurate nu and argp calculation. 
  % Consider using external libraries or implementing them yourself.
  %warning('Elliptical orbit support not implemented. nu and argp might be inaccurate.');
%nu = atan2(r(2), r(1));
end

== matlab function system_model/MATLAB Function1 ==
  data: r input; a output; v input; mu input; e output; i output; Omega output; omega output; nu output
function [a, e, i, Omega, omega, nu] = cart2kep(r, v, mu)
% CART2KEP converts Cartesian coordinates to Keplerian orbital elements
% Input arguments:
% r   - position vector (km)
% v   - velocity vector (km/s)
% mu  - gravitational parameter (km^3/s^2)
% Output arguments:
% a     - semi-major axis (km)
% e     - eccentricity
% i     - inclination (rad)
% Omega - right ascension of the ascending node (rad)
% omega - argument of perigee (rad)
% E     - eccentric anomaly (rad)

% Compute specific angular momentum and its magnitude
h = cross(r, v);
hmag = norm(h);

% Compute semi-latus rectum and eccentricity
rp = hmag^2/mu;
evec = cross(v, h)/mu - r/norm(r);
e = norm(evec);

% Compute semi-major axis and true anomaly
a = rp/(1-e^2);
cos_nu = dot(evec, r)/(e*norm(r));
sin_nu = dot(cross(r, v), h)/(e*norm(r)*hmag);
%nu = atan2(sin_nu, cos_nu);
 % For elliptical orbits, iterative methods like universal variable method 
  % are needed for accurate nu and argp calculation. 
  % Consider using external libraries or implementing them yourself.
  %warning('Elliptical orbit support not implemented. nu and argp might be inaccurate.');
  nu = atan2(r(2), r(1));
% Compute inclination and right ascension of the ascending node
i = acos(h(3)/hmag);
Omega = atan2(h(1), -h(2));

% Compute argument of perigee and eccentric anomaly
cos_omega = evec(1)/e;
sin_omega = evec(2)/e;
omega = atan2(sin_omega, cos_omega);
cos_E = (1 - norm(r)/a)/e;
sin_E = dot(r, v)/(e*norm(r));
E = atan2(sin_E, cos_E);
end

== matlab function system_model/Attitude dynamics/Attitude leader/MATLAB Eq ==
  data: q input; E_q output
function E_q = Eq(q)
      E_q = [q(4)  -q(3)   q(2);
             q(3)   q(4)  -q(1);
            -q(2)   q(1)   q(4);
            -q(1)  -q(2)  -q(3)];

== matlab function system_model/Attitude dynamics/Attitude leader/MATLAB Eq1 ==
  data: q input; E_q output
function E_q = Eq(q)
      E_q = [q(4)  -q(3)   q(2);
             q(3)   q(4)  -q(1);
            -q(2)   q(1)   q(4);
            -q(1)  -q(2)  -q(3)];

== matlab function system_model/Attitude dynamics/MATLAB Function2 ==
  data: B_l output; B_l input; B_f output; B_f input; m_f input; m_l input; B_f_max input; B_l_max input; B_f_min input; theta_l_d output; theta_f_d output; B_l_min input
function [B_l, B_f, theta_l_d, theta_f_d] = ballistic_to_theta(B_l, B_f, m_f, m_l, B_f_max, B_l_max, B_f_min, B_l_min)
%DRAGTOATTITUDE Summary of this function goes here
%   Detailed explanation goes here
% 
% C_d = 2.5;
% C_d_l = C_d;
% C_d_f = C_d;

%Polinomial that represents A_ref*C_d at theta [0.pi/2]
%p = [40.01, -411.74, 327.3, 1173.96, 261.12];
    %p  = [0.00400120687442500	-0.0411735422456600	0.0327337954545250	0.117396192785134	-0.0678880815497270];
    p  = [0.00400120687442530	-0.0411735422456601	0.0327337954545247	0.117396192785134	0.0261119184502728];
    % B_max = 0.081
    % B_min = 0.0130
    %
    theta_l_d = 0;
    theta_f_d = 0;

%Seperate function based on sign of rel_accel

   % B_l = (A_l_min*C_d_l)/ m_l; % must be updated to include the spesific drag coefficent at C_d_0
    
    %B_f = abs(u) + B_l;
    if B_f > B_f_max
        B_f = B_f_max;
    end
    if B_l > B_l_max
        B_l = B_l_max;
    end
    
    Cd_x_A_f = B_f * m_f; % inverse Ballistic coefficent
    % find pitch angle from Cd_x_A_f
    p(5) = p(5) - Cd_x_A_f; % move root to f(theta) = cd_x_A_f
    r = roots(p);
    theta_f_d = select_root(r, 0, pi/2);

    %B_f = (A_f_min*C_d_f)/m_f; % must be updated to include the spesific drag coefficent at C_d_0
    
    %B_l = abs(u) + B_f;
    %p  = [0.00400120687442500	-0.0411735422456600	0.0327337954545250	0.117396192785134	-0.0678880815497270];
    p  = [0.00400120687442530	-0.0411735422456601	0.0327337954545247	0.117396192785134	0.0261119184502728];
    Cd_x_A_l = B_l * m_l; % Inverse ballistic coefficent
    % find pitch angle from Cd_x_A_l
    p(5) = p(5) - Cd_x_A_l; % move root to f(theta) = cd_x_A_f
    r = roots(p);
    theta_l_d = select_root(r, 0, pi/2);

    
end


function root = select_root(roots, lower_bound, upper_bound)
    %extract values that are within the inteval
    root = [];
    sz = size(roots,1);
    for row = 1:sz
        val = roots(row);
        if val > lower_bound && val < upper_bound && imag(val) < 0.01 %isreal( val )
            root(end+1) = real(val);
        end

    end
    if size(root,2) > 1 %( size(root)[2] > 1 )
        %root_index = min(root);
        root = min(root);
        %root = root(root_index);
    end
    
    %sz = size(root,2);
    if size(root,2) < 1
        root = 0; % if no suitable root is found, then the angle could be assumed to be 0 deg
    end
    temp = root(1);
    root = temp;

end
